simulink model "MWT_model_simulink"  (R2021a)
settings: Solver=VariableStepAuto  StartTime=0.0  StopTime=700  RelTol=1e-3
values from neighbouring files (symbols this model uses):
  p = 1.225    [MWT_model_input.m]
  R = 0.75    [MWT_model_input.m]
  Vm = 3    [MWT_model_input.m]
undefined symbols (not defined in the file or in its folder): Me, N, r, sigbuilder_block, wc
libraries: simulink x1, autolibsharedcoupling x1
settings Model: Creator=alevl  LastModifiedBy=alevl

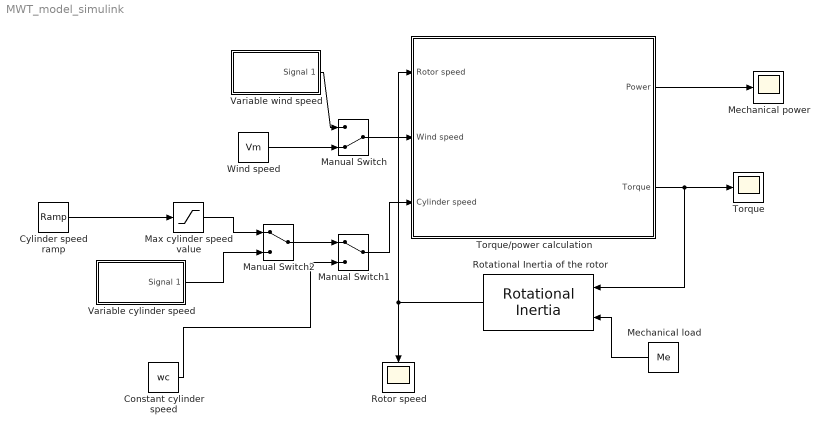
== system MWT_model_simulink ==
  Constant cylinder speed : Constant  Value=wc
  Cylinder speed ramp : simulink/Sources/Ramp  slope=1  start=0  InitialOutput=0
  Manual Switch : ManualSwitch  CurrentSetting=0
  Manual Switch1 : ManualSwitch
  Manual Switch2 : ManualSwitch
  Max cylinder speed value : Saturate  UpperLimit=wc
  Mechanical load : Constant  Value=Me
  Mechanical power : Scope
  Rotational Inertia of the rotor : autolibsharedcoupling/Rotational Inertia  port_config=Simulink  extInfo=off  externJ=off  J=2  b=1.4  omega_o=0.001  blkID=0  aMode=2
      settings: SourceProductBaseCode=PW,DR,MT,UV,VE
  Rotor speed : Scope
  Torque : Scope
  Torque/power calculation : Subsystem
      mask Display: image('C:\Users\alevl\OneDrive\phd\диссер\Assembly_2019-Oct-28_08-08-52PM-000_CustomizedView17615464679.png'); % Use "Edit Image" on toolstrip to change.
  Variable cylinder speed : Subsystem  Tag=STV Subsys  LoadFcn=sigbuilder_block('load');  StartFcn=sigbuilder_block('start');  StopFcn=sigbuilder_block('stop');  ClipboardFcn=sigbuilder_block('clipboard');  mask(Sigbuilder block){tuvar=[0:10]}
      mask help: Simulink:masks:SigbuilderBlock_MD
      mask init:
      | if ~strcmp(get_param(bdroot(gcbh),'SimulationStatus'),'stopped') tuvar = sigbuilder_block('maskInit'); end
      settings: CopyFcn=sigbuilder_block('copy');  DeleteFcn=sigbuilder_block('delete');  ModelCloseFcn=sigbuilder_block('modelClose');  PreSaveFcn=sigbuilder_block('preSave');  PauseFcn=sigbuilder_block('pause');  ContinueFcn=sigbuilder_block('continue');  NameChangeFcn=sigbuilder_block('namechange');  OpenFcn=sigbuilder_block('open',[370.2 159.6 550.8 400.2 ]);  CloseFcn=sigbuilder_block('close');
      mask Display: plot(0, 0, 100, 100,[2, 2, 32, 32, 2], [68, 8, 8, 68, 68],[32, 2], [38, 38], [32, 19, 2],[53, 60, 44], [32, 17, 17, 2],[16, 16, 31, 31]);txt = getActiveGroup(gcbh);text(2, 100, txt,'verticalAlignment', 'top');
  Variable wind speed : Subsystem  Tag=STV Subsys  LoadFcn=sigbuilder_block('load');  StartFcn=sigbuilder_block('start');  StopFcn=sigbuilder_block('stop');  ClipboardFcn=sigbuilder_block('clipboard');  mask(Sigbuilder block){tuvar=[0:10]}
      mask help: Simulink:masks:SigbuilderBlock_MD
      mask init:
      | if ~strcmp(get_param(bdroot(gcbh),'SimulationStatus'),'stopped') tuvar = sigbuilder_block('maskInit'); end
      settings: CopyFcn=sigbuilder_block('copy');  DeleteFcn=sigbuilder_block('delete');  ModelCloseFcn=sigbuilder_block('modelClose');  PreSaveFcn=sigbuilder_block('preSave');  PauseFcn=sigbuilder_block('pause');  ContinueFcn=sigbuilder_block('continue');  NameChangeFcn=sigbuilder_block('namechange');  OpenFcn=sigbuilder_block('open',[370.2 159.6 550.8 400.2 ]);  CloseFcn=sigbuilder_block('close');
      mask Display: plot(0, 0, 100, 100,[2, 2, 32, 32, 2], [68, 8, 8, 68, 68],[32, 2], [38, 38], [32, 19, 2],[53, 60, 44], [32, 17, 17, 2],[16, 16, 31, 31]);txt = getActiveGroup(gcbh);text(2, 100, txt,'verticalAlignment', 'top');
  Wind speed : Constant  Value=Vm
  wires:
  Torque/power calculation/2(Torque) -> Rotational Inertia of the rotor/1, Torque/1
  Torque/power calculation/1(Power) -> Mechanical power/1
  Rotational Inertia of the rotor/1 -> Torque/power calculation/1(Rotor speed), Rotor speed/1
  Wind speed/1 -> Manual Switch/2
  Variable wind speed/1(Signal 1) -> Manual Switch/1
  Manual Switch/1 -> Torque/power calculation/2(Wind speed)
  Cylinder speed ramp/1 -> Max cylinder speed value/1
  Constant cylinder speed/1 -> Manual Switch1/2
  Manual Switch1/1 -> Torque/power calculation/3(Cylinder speed)
  Mechanical load/1 -> Rotational Inertia of the rotor/2
  Max cylinder speed value/1 -> Manual Switch2/1
  Manual Switch2/1 -> Manual Switch1/1
  Variable cylinder speed/1(Signal 1) -> Manual Switch2/2

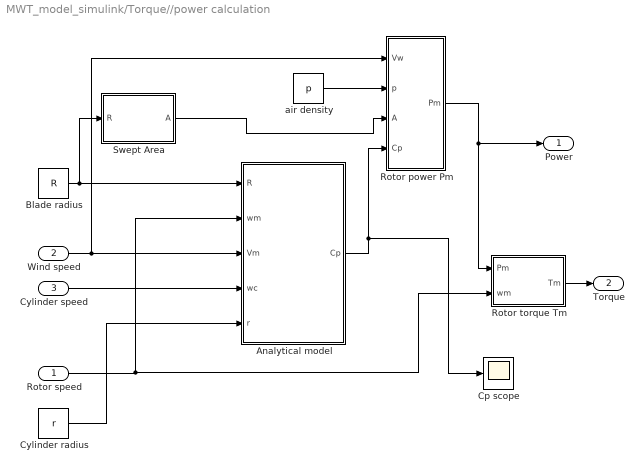
== system MWT_model_simulink/Torque//power calculation ==
  Rotor speed : Inport
  Wind speed : Inport  Port=2
  Cylinder speed : Inport  Port=3
  Analytical model : Subsystem
  Blade radius : Constant  Value=R
  Cp scope : Scope
  Cylinder radius : Constant  Value=r
  Rotor power Pm : MATLAB Function  TreatAsAtomicUnit=on
  Rotor torque Tm : MATLAB Function  TreatAsAtomicUnit=on
  Swept Area : MATLAB Function  TreatAsAtomicUnit=on
  air density : Constant  Value=p
  Power : Outport
  Torque : Outport  Port=2
  wires:
  Analytical model/1(Cp) -> Rotor power Pm/4(Cp), Cp scope/1
  Rotor speed/1 -> Analytical model/2(wm), Rotor torque Tm/2(wm)
  Wind speed/1 -> Rotor power Pm/1(Vw), Analytical model/3(Vm)
  Swept Area/1(A) -> Rotor power Pm/3(A)
  air density/1 -> Rotor power Pm/2(p)
  Blade radius/1 -> Analytical model/1(R), Swept Area/1(R)
  Rotor torque Tm/1(Tm) -> Torque/1
  Rotor power Pm/1(Pm) -> Power/1, Rotor torque Tm/1(Pm)
  Cylinder radius/1 -> Analytical model/5(r)
  Cylinder speed/1 -> Analytical model/4(wc)

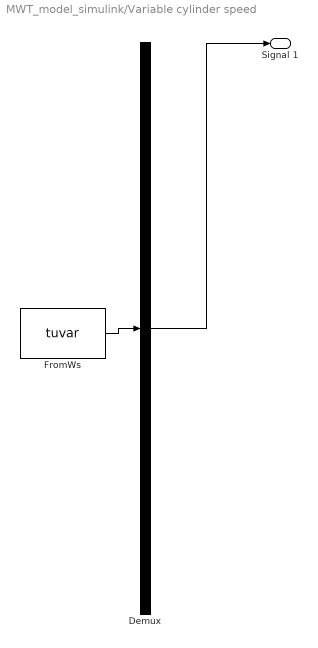
== system MWT_model_simulink/Variable cylinder speed ==
  Demux : Demux  Tag=STV Demux  Outputs=1
      settings: DisplayOption=none
  FromWs : FromWorkspace  Tag=STV FromWs  VariableName=tuvar
      SigBuilderData=|
      | common.afterFinalStr = 'Extrapolate'
      | common.sampleTime = 0
      | dataSet.timeRange = [0 600]
      | dataSet.name = 'Group 1'
      | sbobj.Groups.Name = 'Group 1'
      | sbobj.Groups.Signals.Name = 'Signal 1'
      | sbobj.Groups.Signals.XData = [0 60 60 300 300 540 540 600]
      | sbobj.Groups.Signals.YData = [3 3 15 15 10 10 3 3]
      | sbobj.Groups.TimeRange = [0 600]
  Signal 1 : Outport  Tag=STV Outport
  wires:
  FromWs/1 -> Demux/1
  Demux/1 -> Signal 1/1

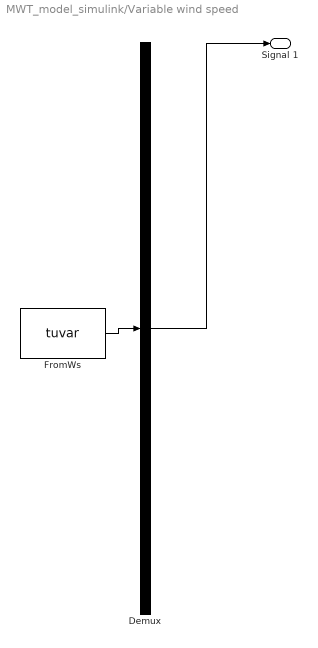
== system MWT_model_simulink/Variable wind speed ==
  Demux : Demux  Tag=STV Demux  Outputs=1
      settings: DisplayOption=none
  FromWs : FromWorkspace  Tag=STV FromWs  VariableName=tuvar
      SigBuilderData=|
      | common.afterFinalStr = 'Extrapolate'
      | common.sampleTime = 0
      | dataSet.timeRange = [0 600]
      | dataSet.name = 'Group 1'
      | sbobj.Groups.Name = 'Group 1'
      | sbobj.Groups.Signals.Name = 'Signal 1'
      | sbobj.Groups.Signals.XData = [0 60 60 300 300 540 540 600]
      | sbobj.Groups.Signals.YData = [3 3 15 15 10 10 3 3]
      | sbobj.Groups.TimeRange = [0 600]
  Signal 1 : Outport  Tag=STV Outport
  wires:
  FromWs/1 -> Demux/1
  Demux/1 -> Signal 1/1

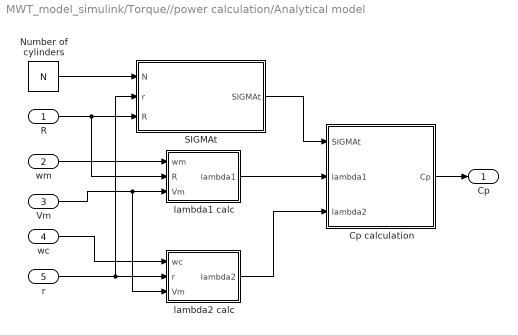
== system MWT_model_simulink/Torque//power calculation/Analytical model ==
  R : Inport
  wm : Inport  Port=2
  Vm : Inport  Port=3
  wc : Inport  Port=4
  r : Inport  Port=5
  Cp calculation : MATLAB Function  TreatAsAtomicUnit=on
  Number of cylinders : Constant  Value=N
  SIGMAt : MATLAB Function  TreatAsAtomicUnit=on
  lambda1 calc : MATLAB Function  TreatAsAtomicUnit=on
  lambda2 calc : MATLAB Function  TreatAsAtomicUnit=on
  Cp : Outport
  wires:
  Number of cylinders/1 -> SIGMAt/1(N)
  lambda1 calc/1(lambda1) -> Cp calculation/2(lambda1)
  wc/1 -> lambda2 calc/1(wc)
  lambda2 calc/1(lambda2) -> Cp calculation/3(lambda2)
  R/1 -> lambda1 calc/2(R), SIGMAt/3(R)
  Cp calculation/1(Cp) -> Cp/1
  SIGMAt/1(SIGMAt) -> Cp calculation/1(SIGMAt)
  wm/1 -> lambda1 calc/1(wm)
  Vm/1 -> lambda2 calc/3(Vm), lambda1 calc/3(Vm)
  r/1 -> SIGMAt/2(r), lambda2 calc/2(r)

== matlab function MWT_model_simulink/Torque//power calculation/Analytical model/lambda1 calc ==
  data: wm input; lambda1 output; R input; Vm input
function lambda1 = fcn(wm,R,Vm)

lambda1 = wm*R/Vm;

== matlab function MWT_model_simulink/Torque//power calculation/Analytical model/lambda2 calc ==
  data: wc input; lambda2 output; r input; Vm input
function lambda2 = fcn(wc,r,Vm)

lambda2 = wc*r/Vm;

== matlab function MWT_model_simulink/Torque//power calculation/Analytical model/Cp calculation ==
  data: SIGMAt input; Cp output; lambda1 input; lambda2 input
function Cp = fcn(SIGMAt,lambda1, lambda2)

Cp = (pi*SIGMAt*lambda1*lambda2)/2*(1+sqrt(1-pi*SIGMAt*lambda1*lambda2));

== matlab function MWT_model_simulink/Torque//power calculation/Analytical model/SIGMAt ==
  data: N input; SIGMAt output; r input; R input
function SIGMAt = fcn(N,r,R)

SIGMAt = 2*N*r/(2*pi*R);

== matlab function MWT_model_simulink/Torque//power calculation/Rotor power Pm ==
  data: Vw input; Pm output; p input; A input; Cp input
function Pm = fcn(Vw,p,A,Cp)

Pm = 1/2*Cp*p*A*Vw^3;

== matlab function MWT_model_simulink/Torque//power calculation/Swept Area ==
  data: R input; A output
function A = fcn(R)

A = R^2*pi;

== matlab function MWT_model_simulink/Torque//power calculation/Rotor torque Tm ==
  data: Pm input; Tm output; wm input
function Tm = fcn(Pm,wm)

Tm = Pm/wm;
